simulink model "CF017A_GmVehPwrMod"  (R2013b)
settings: Solver=FixedStepDiscrete  SolverMode=SingleTasking  StartTime=0.0  StopTime=1  FixedStep=0.002  RelTol=1e-3
values from neighbouring files (symbols this model uses):
  ASSIKEEPMINIDX_CNT_U16 = DataDict.Constant    [CF017A_GmVehPwrMod_DataDict.m]
  BUSOFFHISPDIDX_CNT_U16 = DataDict.Constant    [CF017A_GmVehPwrMod_DataDict.m]
  CNTTOSEC_ULS_U32 = DataDict.Constant    [CF017A_GmVehPwrMod_DataDict.m]
  ENGRUNACTVIDX_CNT_U16 = DataDict.Constant    [CF017A_GmVehPwrMod_DataDict.m]
  GmVehPwrModHwTqMinKeepAssi = DataDict.Calibration    [CF017A_GmVehPwrMod_DataDict.m]
  GmVehPwrModHwTqMinKeepTmr = DataDict.Calibration    [CF017A_GmVehPwrMod_DataDict.m]
  GmVehPwrModOperRampRate = DataDict.Calibration    [CF017A_GmVehPwrMod_DataDict.m]
  GMVEHPWRMODSYSSTREQENA_CNT_LOGL = DataDict.Constant    [CF017A_GmVehPwrMod_DataDict.m]
  GMVEHPWRMODVAREFF_CNT_LOGL = DataDict.Constant    [CF017A_GmVehPwrMod_DataDict.m]
  GmVehPwrModVehSpdAssiOnMin = DataDict.Calibration    [CF017A_GmVehPwrMod_DataDict.m]
  GmVehPwrModVehSpdMinKeepAssi = DataDict.Calibration    [CF017A_GmVehPwrMod_DataDict.m]
  GPIOMCUENAIDX_CNT_U16 = DataDict.Constant    [CF017A_GmVehPwrMod_DataDict.m]
  KEEPASSIIDX_CNT_U16 = DataDict.Constant    [CF017A_GmVehPwrMod_DataDict.m]
  PRPNSYSACTVMSGINVLDIDX_CNT_U16 = DataDict.Constant    [CF017A_GmVehPwrMod_DataDict.m]
  SYSPWRMODMSGINVLDIDX_CNT_U16 = DataDict.Constant    [CF017A_GmVehPwrMod_DataDict.m]
  SYSPWRMODRUNIDX_CNT_U16 = DataDict.Constant    [CF017A_GmVehPwrMod_DataDict.m]
  VEHSPDSNSRVLDIDX_CNT_U16 = DataDict.Constant    [CF017A_GmVehPwrMod_DataDict.m]
libraries: simulink x2, NxtrLim x2, NxtrAbslt x1
(part 3 of 4)

== system CF017A_GmVehPwrMod/GmVehPwrMod/GmVehPwrModPer1/SysStReqEna_LookupTbl_KeepOn_OnToOff/EngRunActv_Bit6 ==
  In1 : Inport  RequirementInfo="{'linktype_rmi_doors' '0000c6e5 (/GM T1XX/SubSystem Specifications/Customer Functions/CF017A GM Vehicle Power Mode)' '#CF017A_114' 'true' 'REQ:  CF017A_114' '' } %GIDa_9dd018ca_3e31_4c4a_90e0_a6ac76f1343b"
  Bit6_0 : Subsystem  RequirementInfo="{'linktype_rmi_doors' '0000c6e5 (/GM T1XX/SubSystem Specifications/Customer Functions/CF017A GM Vehicle Power Mode)' '#CF017A_114' 'true' 'REQ:  CF017A_114' '' } %GIDa_625130ff_287d_43aa_9d60_330dce0521fa"  TreatAsAtomicUnit=on
  Bit6_64 : Subsystem  RequirementInfo="{'linktype_rmi_doors' '0000c6e5 (/GM T1XX/SubSystem Specifications/Customer Functions/CF017A GM Vehicle Power Mode)' '#CF017A_114' 'true' 'REQ:  CF017A_114' '' } %GIDa_af33270b_28d4_422a_b500_86faa96af759"  TreatAsAtomicUnit=on
  CopyRight2 : Subsystem  Description=|  mask(Copyright Information){none=on}
      | Copyright info block.                                               
      |                                                                     
      | Place copyright information at the top of every subsystem in design.
      mask prompts: none "No parameters"
      mask help: Place copyright information at the top of every subsystem in design.
      mask Display:
      | NxtrConf = 'Nexteer Confidential';
      | 
      | sys = bdroot; %handle for the current model ("system")
      | first = get_param(sys,'Created');
      | if(isempty(first))
      |     first = datestr(now,'yyyy');
      | else
      |     first = first(end-3:end);  %year is last four digits
      | end
      | 
      | last = get_param(sys,'LastModifiedDate');
      | if isempty(last)
      |     last = datestr(now,'yyyy');
      | else
      |     last = last(end-3:end);
      | end
      | 
      | if strcmp(first,last)
      |     fprintf('%s -- Copyright %s Nexteer',NxtrConf,first)
      | else
      |     fprintf('%s -- %s%s- %s Nexteer',NxtrConf,char(169),first,last)
      | end
  EngRunActv_IF : If  RequirementInfo="{'linktype_rmi_doors' '0000c6e5 (/GM T1XX/SubSystem Specifications/Customer Functions/CF017A GM Vehicle Power Mode)' '#CF017A_114' 'true' 'REQ:  CF017A_114' '' } %GIDa_4bc83484_183b_4007_801b_23b2c8241593"  IfExpression=u1
  Merge2 : Merge  RequirementInfo="{'linktype_rmi_doors' '0000c6e5 (/GM T1XX/SubSystem Specifications/Customer Functions/CF017A GM Vehicle Power Mode)' '#CF017A_114' 'true' 'REQ:  CF017A_114' '' } %GIDa_7048c8b7_9ac1_4109_96fa_021c302b5bde"
  Out1 : Outport  RequirementInfo="{'linktype_rmi_doors' '0000c6e5 (/GM T1XX/SubSystem Specifications/Customer Functions/CF017A GM Vehicle Power Mode)' '#CF017A_114' 'true' 'REQ:  CF017A_114' '' } %GIDa_5ffbc119_3c40_4564_a8d9_386f6fb67804"
  wires:
  In1/1 -> EngRunActv_IF/1
  EngRunActv_IF/1 -> Bit6_64/Action
  EngRunActv_IF/2 -> Bit6_0/Action
  Bit6_64/1(Bit6Sts) -> Merge2/1
  Bit6_0/1(Bit6Sts) -> Merge2/2
  Merge2/1 -> Out1/1

== system CF017A_GmVehPwrMod/GmVehPwrMod/GmVehPwrModPer1/SysStReqEna_LookupTbl_KeepOn_OnToOff/GpioMcuEna_Bit8 ==
  In : Inport  RequirementInfo="{'linktype_rmi_doors' '0000c6e5 (/GM T1XX/SubSystem Specifications/Customer Functions/CF017A GM Vehicle Power Mode)' '#CF017A_114' 'true' 'REQ:  CF017A_114' '' } %GIDa_b2d8aade_f5d0_444a_a063_7a0289bf908d"
  Bit8_0 : Subsystem  RequirementInfo="{'linktype_rmi_doors' '0000c6e5 (/GM T1XX/SubSystem Specifications/Customer Functions/CF017A GM Vehicle Power Mode)' '#CF017A_114' 'true' 'REQ:  CF017A_114' '' } %GIDa_98c494f0_6c2c_4ada_a798_589724dbf92f"  TreatAsAtomicUnit=on
  Bit8_256 : Subsystem  RequirementInfo="{'linktype_rmi_doors' '0000c6e5 (/GM T1XX/SubSystem Specifications/Customer Functions/CF017A GM Vehicle Power Mode)' '#CF017A_114' 'true' 'REQ:  CF017A_114' '' } %GIDa_a5e75daa_1c3b_4b0f_b862_b737ac528363"  TreatAsAtomicUnit=on
  CopyRight2 : Subsystem  Description=|  mask(Copyright Information){none=on}
      | Copyright info block.                                               
      |                                                                     
      | Place copyright information at the top of every subsystem in design.
      mask prompts: none "No parameters"
      mask help: Place copyright information at the top of every subsystem in design.
      mask Display:
      | NxtrConf = 'Nexteer Confidential';
      | 
      | sys = bdroot; %handle for the current model ("system")
      | first = get_param(sys,'Created');
      | if(isempty(first))
      |     first = datestr(now,'yyyy');
      | else
      |     first = first(end-3:end);  %year is last four digits
      | end
      | 
      | last = get_param(sys,'LastModifiedDate');
      | if isempty(last)
      |     last = datestr(now,'yyyy');
      | else
      |     last = last(end-3:end);
      | end
      | 
      | if strcmp(first,last)
      |     fprintf('%s -- Copyright %s Nexteer',NxtrConf,first)
      | else
      |     fprintf('%s -- %s%s- %s Nexteer',NxtrConf,char(169),first,last)
      | end
  GpioMcuEna_IF : If  RequirementInfo="{'linktype_rmi_doors' '0000c6e5 (/GM T1XX/SubSystem Specifications/Customer Functions/CF017A GM Vehicle Power Mode)' '#CF017A_114' 'true' 'REQ:  CF017A_114' '' } %GIDa_c15d6b31_07d4_4da5_92f4_eebbb80e631b"  IfExpression=u1
  Merge : Merge  RequirementInfo="{'linktype_rmi_doors' '0000c6e5 (/GM T1XX/SubSystem Specifications/Customer Functions/CF017A GM Vehicle Power Mode)' '#CF017A_114' 'true' 'REQ:  CF017A_114' '' } %GIDa_7ac9840a_6a47_4d26_9edd_f2dafb33ce57"
  Out : Outport  RequirementInfo="{'linktype_rmi_doors' '0000c6e5 (/GM T1XX/SubSystem Specifications/Customer Functions/CF017A GM Vehicle Power Mode)' '#CF017A_114' 'true' 'REQ:  CF017A_114' '' } %GIDa_ea86f811_2d4e_4aa3_b284_a4169a7d690f"
  wires:
  In/1 -> GpioMcuEna_IF/1
  GpioMcuEna_IF/1 -> Bit8_256/Action
  GpioMcuEna_IF/2 -> Bit8_0/Action
  Bit8_256/1(Bit8Sts) -> Merge/1
  Bit8_0/1(Bit8Sts) -> Merge/2
  Merge/1 -> Out/1

== system CF017A_GmVehPwrMod/GmVehPwrMod/GmVehPwrModPer1/SysStReqEna_LookupTbl_KeepOn_OnToOff/KeepAssi_Bit0 ==
  In1 : Inport  RequirementInfo="{'linktype_rmi_doors' '0000c6e5 (/GM T1XX/SubSystem Specifications/Customer Functions/CF017A GM Vehicle Power Mode)' '#CF017A_114' 'true' 'REQ:  CF017A_114' '' } %GIDa_256cbed8_1791_4f67_b60a_bd14ae39a67f"
  Bit0_0 : Subsystem  RequirementInfo="{'linktype_rmi_doors' '0000c6e5 (/GM T1XX/SubSystem Specifications/Customer Functions/CF017A GM Vehicle Power Mode)' '#CF017A_114' 'true' 'REQ:  CF017A_114' '' } %GIDa_151fd744_2109_4663_a40c_7bcc314cfd30"  TreatAsAtomicUnit=on
  Bit0_1 : Subsystem  RequirementInfo="{'linktype_rmi_doors' '0000c6e5 (/GM T1XX/SubSystem Specifications/Customer Functions/CF017A GM Vehicle Power Mode)' '#CF017A_114' 'true' 'REQ:  CF017A_114' '' } %GIDa_d6091671_229f_4d66_b3ca_8a783b9b5da7"  TreatAsAtomicUnit=on
  CopyRight2 : Subsystem  Description=|  mask(Copyright Information){none=on}
      | Copyright info block.                                               
      |                                                                     
      | Place copyright information at the top of every subsystem in design.
      mask prompts: none "No parameters"
      mask help: Place copyright information at the top of every subsystem in design.
      mask Display:
      | NxtrConf = 'Nexteer Confidential';
      | 
      | sys = bdroot; %handle for the current model ("system")
      | first = get_param(sys,'Created');
      | if(isempty(first))
      |     first = datestr(now,'yyyy');
      | else
      |     first = first(end-3:end);  %year is last four digits
      | end
      | 
      | last = get_param(sys,'LastModifiedDate');
      | if isempty(last)
      |     last = datestr(now,'yyyy');
      | else
      |     last = last(end-3:end);
      | end
      | 
      | if strcmp(first,last)
      |     fprintf('%s -- Copyright %s Nexteer',NxtrConf,first)
      | else
      |     fprintf('%s -- %s%s- %s Nexteer',NxtrConf,char(169),first,last)
      | end
  KeepAssi_IF : If  RequirementInfo="{'linktype_rmi_doors' '0000c6e5 (/GM T1XX/SubSystem Specifications/Customer Functions/CF017A GM Vehicle Power Mode)' '#CF017A_114' 'true' 'REQ:  CF017A_114' '' } %GIDa_0f92cfb0_47d9_40b4_bb82_e6a253e207e0"  IfExpression=u1
  Merge8 : Merge  RequirementInfo="{'linktype_rmi_doors' '0000c6e5 (/GM T1XX/SubSystem Specifications/Customer Functions/CF017A GM Vehicle Power Mode)' '#CF017A_114' 'true' 'REQ:  CF017A_114' '' } %GIDa_b6c3a93d_a990_4701_9ba0_c730f119e17e"
  Out1 : Outport  RequirementInfo="{'linktype_rmi_doors' '0000c6e5 (/GM T1XX/SubSystem Specifications/Customer Functions/CF017A GM Vehicle Power Mode)' '#CF017A_114' 'true' 'REQ:  CF017A_114' '' } %GIDa_34eb3cf8_5e70_447c_85ff_e4f5d4d1e942"
  wires:
  KeepAssi_IF/1 -> Bit0_1/Action
  KeepAssi_IF/2 -> Bit0_0/Action
  Bit0_1/1(Bit0Sts) -> Merge8/1
  Bit0_0/1(Bit0Sts) -> Merge8/2
  Merge8/1 -> Out1/1
  In1/1 -> KeepAssi_IF/1

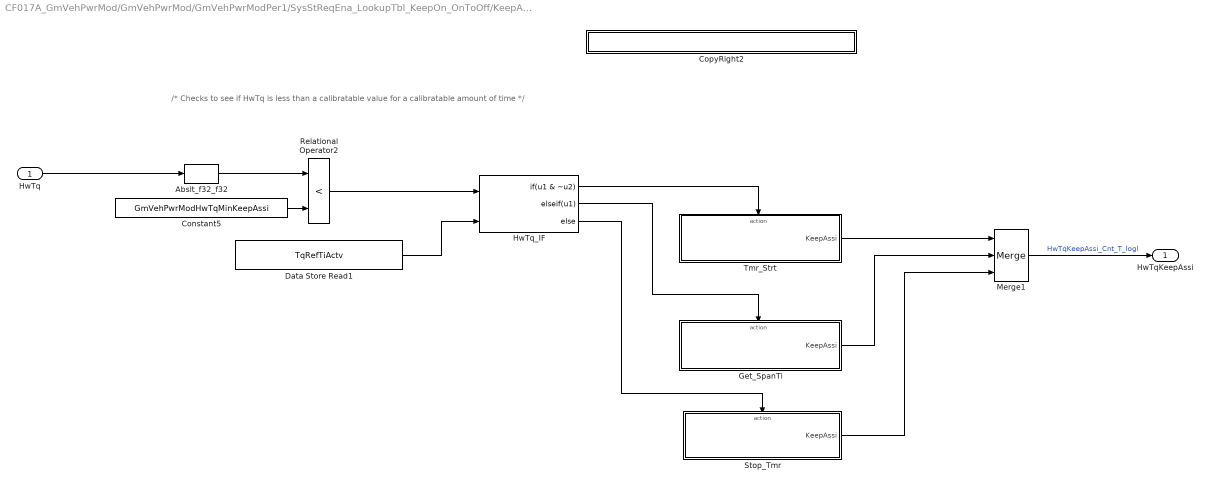
== system CF017A_GmVehPwrMod/GmVehPwrMod/GmVehPwrModPer1/SysStReqEna_LookupTbl_KeepOn_OnToOff/KeepAssi_HwTqTmr ==
  note: /* Checks to see if HwTq is less than a calibratable value for a calibratable amount of time */
  HwTq : Inport  RequirementInfo="{'linktype_rmi_doors' '0000c6e5 (/GM T1XX/SubSystem Specifications/Customer Functions/CF017A GM Vehicle Power Mode)' '#CF017A_114' 'true' 'REQ:  CF017A_114' '' } %GIDa_c3a6937b_df32_440c_ba95_13f74061466f"
  Abslt_f32_f32 : NxtrAbslt/Abslt_f32_f32  RequirementInfo="{'linktype_rmi_doors' '0000c6e5 (/GM T1XX/SubSystem Specifications/Customer Functions/CF017A GM Vehicle Power Mode)' '#CF017A_114' 'true' 'REQ:  CF017A_114' '' } %GIDa_3a5ba81e_d107_4fba_8a7b_6e86486cebbe"  SFunctionSpec=single y1 = Abslt_f32_f32(single u1)
      settings: AttributesFormatString=%<Name>
  Constant5 : Constant  RequirementInfo="{'linktype_rmi_doors' '0000c6e5 (/GM T1XX/SubSystem Specifications/Customer Functions/CF017A GM Vehicle Power Mode)' '#CF017A_114' 'true' 'REQ:  CF017A_114' '' } %GIDa_adffab70_fd73_4ddb_9985_73770c18bc3f"  Value=GmVehPwrModHwTqMinKeepAssi  OutDataTypeStr=single
      settings: AttributesFormatString=%<OutDataTypeStr>
  CopyRight2 : Subsystem  Description=|  mask(Copyright Information){none=on}
      | Copyright info block.                                               
      |                                                                     
      | Place copyright information at the top of every subsystem in design.
      mask prompts: none "No parameters"
      mask help: Place copyright information at the top of every subsystem in design.
      mask Display:
      | NxtrConf = 'Nexteer Confidential';
      | 
      | sys = bdroot; %handle for the current model ("system")
      | first = get_param(sys,'Created');
      | if(isempty(first))
      |     first = datestr(now,'yyyy');
      | else
      |     first = first(end-3:end);  %year is last four digits
      | end
      | 
      | last = get_param(sys,'LastModifiedDate');
      | if isempty(last)
      |     last = datestr(now,'yyyy');
      | else
      |     last = last(end-3:end);
      | end
      | 
      | if strcmp(first,last)
      |     fprintf('%s -- Copyright %s Nexteer',NxtrConf,first)
      | else
      |     fprintf('%s -- %s%s- %s Nexteer',NxtrConf,char(169),first,last)
      | end
  Data Store Read1 : DataStoreRead  RequirementInfo="{'linktype_rmi_doors' '0000c6e5 (/GM T1XX/SubSystem Specifications/Customer Functions/CF017A GM Vehicle Power Mode)' '#CF017A_114' 'true' 'REQ:  CF017A_114' '' } %GIDa_ae007e7c_6e91_4274_8f03_1bad8648c8eb"  DataStoreName=TqRefTiActv
  Get_SpanTi : Subsystem  RequirementInfo="{'linktype_rmi_doors' '0000c6e5 (/GM T1XX/SubSystem Specifications/Customer Functions/CF017A GM Vehicle Power Mode)' '#CF017A_114' 'true' 'REQ:  CF017A_114' '' } %GIDa_763799e1_0442_4180_996d_ddc443fffa17"  TreatAsAtomicUnit=on
  HwTq_IF : If  RequirementInfo="{'linktype_rmi_doors' '0000c6e5 (/GM T1XX/SubSystem Specifications/Customer Functions/CF017A GM Vehicle Power Mode)' '#CF017A_114' 'true' 'REQ:  CF017A_114' '' } %GIDa_62e46df0_927c_4046_91d3_c5bf11f90563"  NumInputs=2  IfExpression=u1 & ~u2  ElseIfExpressions=u1
      settings: AttributesFormatString=%<Priority>
  Merge1 : Merge  RequirementInfo="{'linktype_rmi_doors' '0000c6e5 (/GM T1XX/SubSystem Specifications/Customer Functions/CF017A GM Vehicle Power Mode)' '#CF017A_114' 'true' 'REQ:  CF017A_114' '' } %GIDa_e9a2ff01_7d75_46dd_8799_bdc1acdf7b88"  Inputs=3
  Relational Operator2 : RelationalOperator  RequirementInfo="{'linktype_rmi_doors' '0000c6e5 (/GM T1XX/SubSystem Specifications/Customer Functions/CF017A GM Vehicle Power Mode)' '#CF017A_114' 'true' 'REQ:  CF017A_114' '' } %GIDa_baf5e27b_ba36_44dd_ae20_e2eb1b2ebcf4"  Operator=<  OutDataTypeStr=boolean
  Stop_Tmr : Subsystem  RequirementInfo="{'linktype_rmi_doors' '0000c6e5 (/GM T1XX/SubSystem Specifications/Customer Functions/CF017A GM Vehicle Power Mode)' '#CF017A_114' 'true' 'REQ:  CF017A_114' '' } %GIDa_e3c3fd56_8c35_498f_9322_7430b0bab790"  TreatAsAtomicUnit=on
  Tmr_Strt : Subsystem  RequirementInfo="{'linktype_rmi_doors' '0000c6e5 (/GM T1XX/SubSystem Specifications/Customer Functions/CF017A GM Vehicle Power Mode)' '#CF017A_114' 'true' 'REQ:  CF017A_114' '' } %GIDa_1977e5b8_ee04_4209_b22f_32f27427e055"  TreatAsAtomicUnit=on
  HwTqKeepAssi : Outport  RequirementInfo="{'linktype_rmi_doors' '0000c6e5 (/GM T1XX/SubSystem Specifications/Customer Functions/CF017A GM Vehicle Power Mode)' '#CF017A_114' 'true' 'REQ:  CF017A_114' '' } %GIDa_e791da23_25c1_4c1a_9a17_68a71b1c395d"
  wires:
  Merge1/1 -> HwTqKeepAssi/1  "HwTqKeepAssi_Cnt_T_logl"
  HwTq/1 -> Abslt_f32_f32/1
  HwTq_IF/2 -> Get_SpanTi/Action
  Constant5/1 -> Relational Operator2/2
  Data Store Read1/1 -> HwTq_IF/2
  Abslt_f32_f32/1 -> Relational Operator2/1
  HwTq_IF/3 -> Stop_Tmr/Action
  Relational Operator2/1 -> HwTq_IF/1
  HwTq_IF/1 -> Tmr_Strt/Action
  Stop_Tmr/1("KeepAssi ") -> Merge1/3
  Tmr_Strt/1("KeepAssi ") -> Merge1/1
  Get_SpanTi/1("KeepAssi ") -> Merge1/2

== system CF017A_GmVehPwrMod/GmVehPwrMod/GmVehPwrModPer1/SysStReqEna_LookupTbl_KeepOn_OnToOff/PrpnSysActvMsgInvld_Bit4 ==
  In1 : Inport  RequirementInfo="{'linktype_rmi_doors' '0000c6e5 (/GM T1XX/SubSystem Specifications/Customer Functions/CF017A GM Vehicle Power Mode)' '#CF017A_114' 'true' 'REQ:  CF017A_114' '' } %GIDa_2c591430_5888_4c70_8e6c_3841059961a6"
  Bit4_0 : Subsystem  RequirementInfo="{'linktype_rmi_doors' '0000c6e5 (/GM T1XX/SubSystem Specifications/Customer Functions/CF017A GM Vehicle Power Mode)' '#CF017A_114' 'true' 'REQ:  CF017A_114' '' } %GIDa_0caf3abd_580a_4ffc_a4a2_093dd0efe2b5"  TreatAsAtomicUnit=on
  Bit4_16 : Subsystem  RequirementInfo="{'linktype_rmi_doors' '0000c6e5 (/GM T1XX/SubSystem Specifications/Customer Functions/CF017A GM Vehicle Power Mode)' '#CF017A_114' 'true' 'REQ:  CF017A_114' '' } %GIDa_14718cb4_63e4_496f_b47b_8227a685ab2f"  TreatAsAtomicUnit=on
  CopyRight2 : Subsystem  Description=|  mask(Copyright Information){none=on}
      | Copyright info block.                                               
      |                                                                     
      | Place copyright information at the top of every subsystem in design.
      mask prompts: none "No parameters"
      mask help: Place copyright information at the top of every subsystem in design.
      mask Display:
      | NxtrConf = 'Nexteer Confidential';
      | 
      | sys = bdroot; %handle for the current model ("system")
      | first = get_param(sys,'Created');
      | if(isempty(first))
      |     first = datestr(now,'yyyy');
      | else
      |     first = first(end-3:end);  %year is last four digits
      | end
      | 
      | last = get_param(sys,'LastModifiedDate');
      | if isempty(last)
      |     last = datestr(now,'yyyy');
      | else
      |     last = last(end-3:end);
      | end
      | 
      | if strcmp(first,last)
      |     fprintf('%s -- Copyright %s Nexteer',NxtrConf,first)
      | else
      |     fprintf('%s -- %s%s- %s Nexteer',NxtrConf,char(169),first,last)
      | end
  Merge4 : Merge  RequirementInfo="{'linktype_rmi_doors' '0000c6e5 (/GM T1XX/SubSystem Specifications/Customer Functions/CF017A GM Vehicle Power Mode)' '#CF017A_114' 'true' 'REQ:  CF017A_114' '' } %GIDa_4aefb7ab_6048_4fba_b30f_165c5c5a5fc7"
  Msg0C9Missa_IF : If  RequirementInfo="{'linktype_rmi_doors' '0000c6e5 (/GM T1XX/SubSystem Specifications/Customer Functions/CF017A GM Vehicle Power Mode)' '#CF017A_114' 'true' 'REQ:  CF017A_114' '' } %GIDa_4ef6b54c_1cdc_4af6_96da_f9013792689e"  IfExpression=u1
  Out1 : Outport  RequirementInfo="{'linktype_rmi_doors' '0000c6e5 (/GM T1XX/SubSystem Specifications/Customer Functions/CF017A GM Vehicle Power Mode)' '#CF017A_114' 'true' 'REQ:  CF017A_114' '' } %GIDa_0572da8d_4d01_4630_a2fe_8cdb88bfe4d3"
  wires:
  In1/1 -> Msg0C9Missa_IF/1
  Msg0C9Missa_IF/1 -> Bit4_16/Action
  Msg0C9Missa_IF/2 -> Bit4_0/Action
  Bit4_16/1(Bit4Sts) -> Merge4/1
  Bit4_0/1(Bit4Sts) -> Merge4/2
  Merge4/1 -> Out1/1

== system CF017A_GmVehPwrMod/GmVehPwrMod/GmVehPwrModPer1/SysStReqEna_LookupTbl_KeepOn_OnToOff/SysPwrModMsgInvld_Bit2 ==
  In1 : Inport  RequirementInfo="{'linktype_rmi_doors' '0000c6e5 (/GM T1XX/SubSystem Specifications/Customer Functions/CF017A GM Vehicle Power Mode)' '#CF017A_114' 'true' 'REQ:  CF017A_114' '' } %GIDa_b9b4edaa_6008_4e55_867c_388323464606"
  Bit2_0 : Subsystem  RequirementInfo="{'linktype_rmi_doors' '0000c6e5 (/GM T1XX/SubSystem Specifications/Customer Functions/CF017A GM Vehicle Power Mode)' '#CF017A_114' 'true' 'REQ:  CF017A_114' '' } %GIDa_b11557df_5945_49a6_a0af_1b2573475ba6"  TreatAsAtomicUnit=on
  Bit2_4 : Subsystem  RequirementInfo="{'linktype_rmi_doors' '0000c6e5 (/GM T1XX/SubSystem Specifications/Customer Functions/CF017A GM Vehicle Power Mode)' '#CF017A_114' 'true' 'REQ:  CF017A_114' '' } %GIDa_538bca24_1df9_41e8_ac8e_fc9e4c129984"  TreatAsAtomicUnit=on
  CopyRight2 : Subsystem  Description=|  mask(Copyright Information){none=on}
      | Copyright info block.                                               
      |                                                                     
      | Place copyright information at the top of every subsystem in design.
      mask prompts: none "No parameters"
      mask help: Place copyright information at the top of every subsystem in design.
      mask Display:
      | NxtrConf = 'Nexteer Confidential';
      | 
      | sys = bdroot; %handle for the current model ("system")
      | first = get_param(sys,'Created');
      | if(isempty(first))
      |     first = datestr(now,'yyyy');
      | else
      |     first = first(end-3:end);  %year is last four digits
      | end
      | 
      | last = get_param(sys,'LastModifiedDate');
      | if isempty(last)
      |     last = datestr(now,'yyyy');
      | else
      |     last = last(end-3:end);
      | end
      | 
      | if strcmp(first,last)
      |     fprintf('%s -- Copyright %s Nexteer',NxtrConf,first)
      | else
      |     fprintf('%s -- %s%s- %s Nexteer',NxtrConf,char(169),first,last)
      | end
  Merge6 : Merge  RequirementInfo="{'linktype_rmi_doors' '0000c6e5 (/GM T1XX/SubSystem Specifications/Customer Functions/CF017A GM Vehicle Power Mode)' '#CF017A_114' 'true' 'REQ:  CF017A_114' '' } %GIDa_c748d9e6_4e3c_4f18_8982_64515a3432db"
  Msg1F1Miss_IF : If  RequirementInfo="{'linktype_rmi_doors' '0000c6e5 (/GM T1XX/SubSystem Specifications/Customer Functions/CF017A GM Vehicle Power Mode)' '#CF017A_114' 'true' 'REQ:  CF017A_114' '' } %GIDa_7c507352_f8cc_4c21_a6de_4c1245659dbe"  IfExpression=u1
  Out1 : Outport  RequirementInfo="{'linktype_rmi_doors' '0000c6e5 (/GM T1XX/SubSystem Specifications/Customer Functions/CF017A GM Vehicle Power Mode)' '#CF017A_114' 'true' 'REQ:  CF017A_114' '' } %GIDa_11135a2a_4b33_4b18_b28c_32efa3fd628e"
  wires:
  In1/1 -> Msg1F1Miss_IF/1
  Msg1F1Miss_IF/1 -> Bit2_4/Action
  Msg1F1Miss_IF/2 -> Bit2_0/Action
  Bit2_4/1(Bit2Sts) -> Merge6/1
  Bit2_0/1(Bit2Sts) -> Merge6/2
  Merge6/1 -> Out1/1

== system CF017A_GmVehPwrMod/GmVehPwrMod/GmVehPwrModPer1/SysStReqEna_LookupTbl_KeepOn_OnToOff/SysPwrModRun_Bit7 ==
  In1 : Inport  RequirementInfo="{'linktype_rmi_doors' '0000c6e5 (/GM T1XX/SubSystem Specifications/Customer Functions/CF017A GM Vehicle Power Mode)' '#CF017A_114' 'true' 'REQ:  CF017A_114' '' } %GIDa_c1bc1cd8_ea72_4c59_9135_af5cdd5d310f"
  Bit7_0 : Subsystem  RequirementInfo="{'linktype_rmi_doors' '0000c6e5 (/GM T1XX/SubSystem Specifications/Customer Functions/CF017A GM Vehicle Power Mode)' '#CF017A_114' 'true' 'REQ:  CF017A_114' '' } %GIDa_c8c3ffe3_12b8_4e4f_8a91_02b5fec5e3dd"  TreatAsAtomicUnit=on
  Bit7_128 : Subsystem  RequirementInfo="{'linktype_rmi_doors' '0000c6e5 (/GM T1XX/SubSystem Specifications/Customer Functions/CF017A GM Vehicle Power Mode)' '#CF017A_114' 'true' 'REQ:  CF017A_114' '' } %GIDa_e75e24b2_0a88_446a_a5f8_10565f6eaf7b"  TreatAsAtomicUnit=on
  CopyRight2 : Subsystem  Description=|  mask(Copyright Information){none=on}
      | Copyright info block.                                               
      |                                                                     
      | Place copyright information at the top of every subsystem in design.
      mask prompts: none "No parameters"
      mask help: Place copyright information at the top of every subsystem in design.
      mask Display:
      | NxtrConf = 'Nexteer Confidential';
      | 
      | sys = bdroot; %handle for the current model ("system")
      | first = get_param(sys,'Created');
      | if(isempty(first))
      |     first = datestr(now,'yyyy');
      | else
      |     first = first(end-3:end);  %year is last four digits
      | end
      | 
      | last = get_param(sys,'LastModifiedDate');
      | if isempty(last)
      |     last = datestr(now,'yyyy');
      | else
      |     last = last(end-3:end);
      | end
      | 
      | if strcmp(first,last)
      |     fprintf('%s -- Copyright %s Nexteer',NxtrConf,first)
      | else
      |     fprintf('%s -- %s%s- %s Nexteer',NxtrConf,char(169),first,last)
      | end
  Merge1 : Merge  RequirementInfo="{'linktype_rmi_doors' '0000c6e5 (/GM T1XX/SubSystem Specifications/Customer Functions/CF017A GM Vehicle Power Mode)' '#CF017A_114' 'true' 'REQ:  CF017A_114' '' } %GIDa_47a35ad3_3413_4261_bf5c_ed15bdd468af"
  SysPwrModRun_IF : If  RequirementInfo="{'linktype_rmi_doors' '0000c6e5 (/GM T1XX/SubSystem Specifications/Customer Functions/CF017A GM Vehicle Power Mode)' '#CF017A_114' 'true' 'REQ:  CF017A_114' '' } %GIDa_3041b7fe_d5e9_45a7_907b_deaf3c12d1b7"  IfExpression=u1
  Out1 : Outport  RequirementInfo="{'linktype_rmi_doors' '0000c6e5 (/GM T1XX/SubSystem Specifications/Customer Functions/CF017A GM Vehicle Power Mode)' '#CF017A_114' 'true' 'REQ:  CF017A_114' '' } %GIDa_ea562539_c8ee_4d74_8941_942a4f0ad269"
  wires:
  In1/1 -> SysPwrModRun_IF/1
  SysPwrModRun_IF/1 -> Bit7_128/Action
  SysPwrModRun_IF/2 -> Bit7_0/Action
  Bit7_128/1(Bit7Sts) -> Merge1/1
  Bit7_0/1(Bit7Sts) -> Merge1/2
  Merge1/1 -> Out1/1

== system CF017A_GmVehPwrMod/GmVehPwrMod/GmVehPwrModPer1/SysStReqEna_LookupTbl_KeepOn_OnToOff/VehSpdSnsrVld_Bit3 ==
  In1 : Inport  RequirementInfo="{'linktype_rmi_doors' '0000c6e5 (/GM T1XX/SubSystem Specifications/Customer Functions/CF017A GM Vehicle Power Mode)' '#CF017A_114' 'true' 'REQ:  CF017A_114' '' } %GIDa_8aa9f388_a059_4463_8363_1874a8a11e12"
  Bit3_0 : Subsystem  RequirementInfo="{'linktype_rmi_doors' '0000c6e5 (/GM T1XX/SubSystem Specifications/Customer Functions/CF017A GM Vehicle Power Mode)' '#CF017A_114' 'true' 'REQ:  CF017A_114' '' } %GIDa_7ba2b7bb_b741_42b3_bd80_f659c1994e0e"  TreatAsAtomicUnit=on
  Bit3_8 : Subsystem  RequirementInfo="{'linktype_rmi_doors' '0000c6e5 (/GM T1XX/SubSystem Specifications/Customer Functions/CF017A GM Vehicle Power Mode)' '#CF017A_114' 'true' 'REQ:  CF017A_114' '' } %GIDa_fcf82675_d7c2_47d8_9612_37435f26f06f"  TreatAsAtomicUnit=on
  CopyRight2 : Subsystem  Description=|  mask(Copyright Information){none=on}
      | Copyright info block.                                               
      |                                                                     
      | Place copyright information at the top of every subsystem in design.
      mask prompts: none "No parameters"
      mask help: Place copyright information at the top of every subsystem in design.
      mask Display:
      | NxtrConf = 'Nexteer Confidential';
      | 
      | sys = bdroot; %handle for the current model ("system")
      | first = get_param(sys,'Created');
      | if(isempty(first))
      |     first = datestr(now,'yyyy');
      | else
      |     first = first(end-3:end);  %year is last four digits
      | end
      | 
      | last = get_param(sys,'LastModifiedDate');
      | if isempty(last)
      |     last = datestr(now,'yyyy');
      | else
      |     last = last(end-3:end);
      | end
      | 
      | if strcmp(first,last)
      |     fprintf('%s -- Copyright %s Nexteer',NxtrConf,first)
      | else
      |     fprintf('%s -- %s%s- %s Nexteer',NxtrConf,char(169),first,last)
      | end
  Merge5 : Merge  RequirementInfo="{'linktype_rmi_doors' '0000c6e5 (/GM T1XX/SubSystem Specifications/Customer Functions/CF017A GM Vehicle Power Mode)' '#CF017A_114' 'true' 'REQ:  CF017A_114' '' } %GIDa_5fe1fb49_98f0_4faf_b2eb_ad195c38c3fa"
  VehSpdSnsrVld_IF : If  RequirementInfo="{'linktype_rmi_doors' '0000c6e5 (/GM T1XX/SubSystem Specifications/Customer Functions/CF017A GM Vehicle Power Mode)' '#CF017A_114' 'true' 'REQ:  CF017A_114' '' } %GIDa_38f90319_4c08_4272_be31_7c36c1ecbd1c"  IfExpression=u1
  Out1 : Outport  RequirementInfo="{'linktype_rmi_doors' '0000c6e5 (/GM T1XX/SubSystem Specifications/Customer Functions/CF017A GM Vehicle Power Mode)' '#CF017A_114' 'true' 'REQ:  CF017A_114' '' } %GIDa_4d69da4a_8e85_4df4_ba86_5b3d7666622a"
  wires:
  In1/1 -> VehSpdSnsrVld_IF/1
  VehSpdSnsrVld_IF/1 -> Bit3_8/Action
  VehSpdSnsrVld_IF/2 -> Bit3_0/Action
  Bit3_8/1(Bit3Sts) -> Merge5/1
  Bit3_0/1(Bit3Sts) -> Merge5/2
  Merge5/1 -> Out1/1

== system CF017A_GmVehPwrMod/GmVehPwrMod/GmVehPwrModPer1/SysStReqEna_Ovrd/CopyRight2 ==

== system CF017A_GmVehPwrMod/GmVehPwrMod/GmVehPwrModPer1/TqCmdSca_VehSpdEna_Sub/CopyRight2 ==

== system CF017A_GmVehPwrMod/GmVehPwrMod/GmVehPwrModPer1/TqCmdSca_VehSpdEna_Sub/Set_SpdEna_False ==
  Action Port : ActionPort  ActionType=else
  Constant4 : Constant  RequirementInfo={} %GIDa_c969a244_c718_4e47_8c5d_d3e9949f60e3  Value=false  OutDataTypeStr=boolean
      settings: AttributesFormatString=%<OutDataTypeStr>
  CopyRight2 : Subsystem  Description=|  mask(Copyright Information){none=on}
      | Copyright info block.                                               
      |                                                                     
      | Place copyright information at the top of every subsystem in design.
      mask prompts: none "No parameters"
      mask help: Place copyright information at the top of every subsystem in design.
      mask Display:
      | NxtrConf = 'Nexteer Confidential';
      | 
      | sys = bdroot; %handle for the current model ("system")
      | first = get_param(sys,'Created');
      | if(isempty(first))
      |     first = datestr(now,'yyyy');
      | else
      |     first = first(end-3:end);  %year is last four digits
      | end
      | 
      | last = get_param(sys,'LastModifiedDate');
      | if isempty(last)
      |     last = datestr(now,'yyyy');
      | else
      |     last = last(end-3:end);
      | end
      | 
      | if strcmp(first,last)
      |     fprintf('%s -- Copyright %s Nexteer',NxtrConf,first)
      | else
      |     fprintf('%s -- %s%s- %s Nexteer',NxtrConf,char(169),first,last)
      | end
  "VehPwrModDftVehSpdEna " : Outport  RequirementInfo={} %GIDa_8e8bb61c_0665_4633_a294_c6f31ae58305
  wires:
  Constant4/1 -> "VehPwrModDftVehSpdEna "/1

== system CF017A_GmVehPwrMod/GmVehPwrMod/GmVehPwrModPer1/TqCmdSca_VehSpdEna_Sub/Set_SpdEna_True ==
  Action Port : ActionPort  ActionType=then
  Constant4 : Constant  RequirementInfo={} %GIDa_68d2d2ab_9cf3_4882_b287_021cb7e5d3a2  Value=true  OutDataTypeStr=boolean
      settings: AttributesFormatString=%<OutDataTypeStr>
  CopyRight2 : Subsystem  Description=|  mask(Copyright Information){none=on}
      | Copyright info block.                                               
      |                                                                     
      | Place copyright information at the top of every subsystem in design.
      mask prompts: none "No parameters"
      mask help: Place copyright information at the top of every subsystem in design.
      mask Display:
      | NxtrConf = 'Nexteer Confidential';
      | 
      | sys = bdroot; %handle for the current model ("system")
      | first = get_param(sys,'Created');
      | if(isempty(first))
      |     first = datestr(now,'yyyy');
      | else
      |     first = first(end-3:end);  %year is last four digits
      | end
      | 
      | last = get_param(sys,'LastModifiedDate');
      | if isempty(last)
      |     last = datestr(now,'yyyy');
      | else
      |     last = last(end-3:end);
      | end
      | 
      | if strcmp(first,last)
      |     fprintf('%s -- Copyright %s Nexteer',NxtrConf,first)
      | else
      |     fprintf('%s -- %s%s- %s Nexteer',NxtrConf,char(169),first,last)
      | end
  "VehPwrModDftVehSpdEna " : Outport  RequirementInfo={} %GIDa_cf3d7fa0_713b_4590_9a5a_32eeb1bd4bc9
  wires:
  Constant4/1 -> "VehPwrModDftVehSpdEna "/1

== system CF017A_GmVehPwrMod/GmVehPwrMod/GmVehPwrModPer1/TqCmdSca_VehSpdEna_Sub/TqCmdSca_0 ==
  Action Port : ActionPort  ActionType=else
  Constant3 : Constant  RequirementInfo="{'linktype_rmi_doors' '0000c6e5 (/GM T1XX/SubSystem Specifications/Customer Functions/CF017A GM Vehicle Power Mode)' '#CF017A_141' 'true' 'REQ:  CF017A_141' '' } %GIDa_6728cc2d_06c9_4a30_b7ce_581745178746"  Value=0  OutDataTypeStr=single
      settings: AttributesFormatString=%<OutDataTypeStr>
  CopyRight2 : Subsystem  Description=|  mask(Copyright Information){none=on}
      | Copyright info block.                                               
      |                                                                     
      | Place copyright information at the top of every subsystem in design.
      mask prompts: none "No parameters"
      mask help: Place copyright information at the top of every subsystem in design.
      mask Display:
      | NxtrConf = 'Nexteer Confidential';
      | 
      | sys = bdroot; %handle for the current model ("system")
      | first = get_param(sys,'Created');
      | if(isempty(first))
      |     first = datestr(now,'yyyy');
      | else
      |     first = first(end-3:end);  %year is last four digits
      | end
      | 
      | last = get_param(sys,'LastModifiedDate');
      | if isempty(last)
      |     last = datestr(now,'yyyy');
      | else
      |     last = last(end-3:end);
      | end
      | 
      | if strcmp(first,last)
      |     fprintf('%s -- Copyright %s Nexteer',NxtrConf,first)
      | else
      |     fprintf('%s -- %s%s- %s Nexteer',NxtrConf,char(169),first,last)
      | end
  SysOperMotTqCmdSca : Outport  RequirementInfo="{'linktype_rmi_doors' '0000c6e5 (/GM T1XX/SubSystem Specifications/Customer Functions/CF017A GM Vehicle Power Mode)' '#CF017A_141' 'true' 'REQ:  CF017A_141' '' } %GIDa_45580eef_5c3d_47bb_8207_d1896df57891"
  wires:
  Constant3/1 -> SysOperMotTqCmdSca/1

== system CF017A_GmVehPwrMod/GmVehPwrMod/GmVehPwrModPer1/TqCmdSca_VehSpdEna_Sub/TqCmdSca_1 ==
  Action Port : ActionPort  ActionType=then
  Constant3 : Constant  RequirementInfo="{'linktype_rmi_doors' '0000c6e5 (/GM T1XX/SubSystem Specifications/Customer Functions/CF017A GM Vehicle Power Mode)' '#CF017A_140' 'true' 'REQ:  CF017A_140' '' } %GIDa_de4d9e3c_2f27_4979_bc11_a6c27cecaf0c"  OutDataTypeStr=single
      settings: AttributesFormatString=%<OutDataTypeStr>
  CopyRight2 : Subsystem  Description=|  mask(Copyright Information){none=on}
      | Copyright info block.                                               
      |                                                                     
      | Place copyright information at the top of every subsystem in design.
      mask prompts: none "No parameters"
      mask help: Place copyright information at the top of every subsystem in design.
      mask Display:
      | NxtrConf = 'Nexteer Confidential';
      | 
      | sys = bdroot; %handle for the current model ("system")
      | first = get_param(sys,'Created');
      | if(isempty(first))
      |     first = datestr(now,'yyyy');
      | else
      |     first = first(end-3:end);  %year is last four digits
      | end
      | 
      | last = get_param(sys,'LastModifiedDate');
      | if isempty(last)
      |     last = datestr(now,'yyyy');
      | else
      |     last = last(end-3:end);
      | end
      | 
      | if strcmp(first,last)
      |     fprintf('%s -- Copyright %s Nexteer',NxtrConf,first)
      | else
      |     fprintf('%s -- %s%s- %s Nexteer',NxtrConf,char(169),first,last)
      | end
  SysOperMotTqCmdSca : Outport  RequirementInfo="{'linktype_rmi_doors' '0000c6e5 (/GM T1XX/SubSystem Specifications/Customer Functions/CF017A GM Vehicle Power Mode)' '#CF017A_140' 'true' 'REQ:  CF017A_140' '' } %GIDa_a7bc3936_d85d_4417_8c6d_43324766451b"
  wires:
  Constant3/1 -> SysOperMotTqCmdSca/1

== system CF017A_GmVehPwrMod/GmVehPwrMod/GmVehPwrModPer1/AssiOnMin_AssiKeepMin/AssiKeepMin_False/CopyRight2 ==

== system CF017A_GmVehPwrMod/GmVehPwrMod/GmVehPwrModPer1/AssiOnMin_AssiKeepMin/AssiKeepMin_True/CopyRight2 ==

== system CF017A_GmVehPwrMod/GmVehPwrMod/GmVehPwrModPer1/AssiOnMin_AssiKeepMin/AssiOnMin_False/CopyRight2 ==

== system CF017A_GmVehPwrMod/GmVehPwrMod/GmVehPwrModPer1/AssiOnMin_AssiKeepMin/AssiOnMin_True/CopyRight2 ==

== system CF017A_GmVehPwrMod/GmVehPwrMod/GmVehPwrModPer1/PwrSplyEnaReq_Sub/PwrSplyEnReq_False/CopyRight2 ==

== system CF017A_GmVehPwrMod/GmVehPwrMod/GmVehPwrModPer1/PwrSplyEnaReq_Sub/PwrSplyEnReq_True/CopyRight2 ==

== system CF017A_GmVehPwrMod/GmVehPwrMod/GmVehPwrModPer1/SysStReqEna_AssiOffToOn/Set_SysStReqEna_False/CopyRight2 ==

== system CF017A_GmVehPwrMod/GmVehPwrMod/GmVehPwrModPer1/SysStReqEna_AssiOffToOn/Set_SysStReqEna_True_Con1/CopyRight2 ==

== system CF017A_GmVehPwrMod/GmVehPwrMod/GmVehPwrModPer1/SysStReqEna_AssiOffToOn/Set_SysStReqEna_True_Con2/CopyRight2 ==

== system CF017A_GmVehPwrMod/GmVehPwrMod/GmVehPwrModPer1/SysStReqEna_LookupTbl_KeepOn_OnToOff/AssiKeepMin_Bit5/Bit5_0 ==
  Action Port : ActionPort  ActionType=else
  Constant2 : Constant  Value=0  OutDataTypeStr=uint16
      settings: AttributesFormatString=%<OutDataTypeStr>
  CopyRight2 : Subsystem  Description=|  mask(Copyright Information){none=on}
      | Copyright info block.                                               
      |                                                                     
      | Place copyright information at the top of every subsystem in design.
      mask prompts: none "No parameters"
      mask help: Place copyright information at the top of every subsystem in design.
      mask Display:
      | NxtrConf = 'Nexteer Confidential';
      | 
      | sys = bdroot; %handle for the current model ("system")
      | first = get_param(sys,'Created');
      | if(isempty(first))
      |     first = datestr(now,'yyyy');
      | else
      |     first = first(end-3:end);  %year is last four digits
      | end
      | 
      | last = get_param(sys,'LastModifiedDate');
      | if isempty(last)
      |     last = datestr(now,'yyyy');
      | else
      |     last = last(end-3:end);
      | end
      | 
      | if strcmp(first,last)
      |     fprintf('%s -- Copyright %s Nexteer',NxtrConf,first)
      | else
      |     fprintf('%s -- %s%s- %s Nexteer',NxtrConf,char(169),first,last)
      | end
  Bit5Sts : Outport
  wires:
  Constant2/1 -> Bit5Sts/1

== system CF017A_GmVehPwrMod/GmVehPwrMod/GmVehPwrModPer1/SysStReqEna_LookupTbl_KeepOn_OnToOff/AssiKeepMin_Bit5/Bit5_32 ==
  Action Port : ActionPort  ActionType=then
  Constant : Constant  Value=ASSIKEEPMINIDX_CNT_U16  OutDataTypeStr=uint16
  CopyRight2 : Subsystem  Description=|  mask(Copyright Information){none=on}
      | Copyright info block.                                               
      |                                                                     
      | Place copyright information at the top of every subsystem in design.
      mask prompts: none "No parameters"
      mask help: Place copyright information at the top of every subsystem in design.
      mask Display:
      | NxtrConf = 'Nexteer Confidential';
      | 
      | sys = bdroot; %handle for the current model ("system")
      | first = get_param(sys,'Created');
      | if(isempty(first))
      |     first = datestr(now,'yyyy');
      | else
      |     first = first(end-3:end);  %year is last four digits
      | end
      | 
      | last = get_param(sys,'LastModifiedDate');
      | if isempty(last)
      |     last = datestr(now,'yyyy');
      | else
      |     last = last(end-3:end);
      | end
      | 
      | if strcmp(first,last)
      |     fprintf('%s -- Copyright %s Nexteer',NxtrConf,first)
      | else
      |     fprintf('%s -- %s%s- %s Nexteer',NxtrConf,char(169),first,last)
      | end
  Bit5Sts : Outport
  wires:
  Constant/1 -> Bit5Sts/1

== system CF017A_GmVehPwrMod/GmVehPwrMod/GmVehPwrModPer1/SysStReqEna_LookupTbl_KeepOn_OnToOff/AssiKeepMin_Bit5/CopyRight2 ==

== system CF017A_GmVehPwrMod/GmVehPwrMod/GmVehPwrModPer1/SysStReqEna_LookupTbl_KeepOn_OnToOff/BusOffHiSpd_Bit1/Bit1_0 ==
  Action Port : ActionPort  ActionType=else
  Constant1 : Constant  Value=0  OutDataTypeStr=uint16
      settings: AttributesFormatString=%<OutDataTypeStr>
  CopyRight2 : Subsystem  Description=|  mask(Copyright Information){none=on}
      | Copyright info block.                                               
      |                                                                     
      | Place copyright information at the top of every subsystem in design.
      mask prompts: none "No parameters"
      mask help: Place copyright information at the top of every subsystem in design.
      mask Display:
      | NxtrConf = 'Nexteer Confidential';
      | 
      | sys = bdroot; %handle for the current model ("system")
      | first = get_param(sys,'Created');
      | if(isempty(first))
      |     first = datestr(now,'yyyy');
      | else
      |     first = first(end-3:end);  %year is last four digits
      | end
      | 
      | last = get_param(sys,'LastModifiedDate');
      | if isempty(last)
      |     last = datestr(now,'yyyy');
      | else
      |     last = last(end-3:end);
      | end
      | 
      | if strcmp(first,last)
      |     fprintf('%s -- Copyright %s Nexteer',NxtrConf,first)
      | else
      |     fprintf('%s -- %s%s- %s Nexteer',NxtrConf,char(169),first,last)
      | end
  Bit1Sts : Outport
  wires:
  Constant1/1 -> Bit1Sts/1

== system CF017A_GmVehPwrMod/GmVehPwrMod/GmVehPwrModPer1/SysStReqEna_LookupTbl_KeepOn_OnToOff/BusOffHiSpd_Bit1/Bit1_2 ==
  Action Port : ActionPort  ActionType=then
  Constant : Constant  Value=BUSOFFHISPDIDX_CNT_U16  OutDataTypeStr=uint16
  CopyRight2 : Subsystem  Description=|  mask(Copyright Information){none=on}
      | Copyright info block.                                               
      |                                                                     
      | Place copyright information at the top of every subsystem in design.
      mask prompts: none "No parameters"
      mask help: Place copyright information at the top of every subsystem in design.
      mask Display:
      | NxtrConf = 'Nexteer Confidential';
      | 
      | sys = bdroot; %handle for the current model ("system")
      | first = get_param(sys,'Created');
      | if(isempty(first))
      |     first = datestr(now,'yyyy');
      | else
      |     first = first(end-3:end);  %year is last four digits
      | end
      | 
      | last = get_param(sys,'LastModifiedDate');
      | if isempty(last)
      |     last = datestr(now,'yyyy');
      | else
      |     last = last(end-3:end);
      | end
      | 
      | if strcmp(first,last)
      |     fprintf('%s -- Copyright %s Nexteer',NxtrConf,first)
      | else
      |     fprintf('%s -- %s%s- %s Nexteer',NxtrConf,char(169),first,last)
      | end
  Bit1Sts : Outport
  wires:
  Constant/1 -> Bit1Sts/1

== system CF017A_GmVehPwrMod/GmVehPwrMod/GmVehPwrModPer1/SysStReqEna_LookupTbl_KeepOn_OnToOff/BusOffHiSpd_Bit1/CopyRight2 ==

== system CF017A_GmVehPwrMod/GmVehPwrMod/GmVehPwrModPer1/SysStReqEna_LookupTbl_KeepOn_OnToOff/EngRunActv_Bit6/Bit6_0 ==
  Action Port : ActionPort  ActionType=else
  Constant1 : Constant  Value=0  OutDataTypeStr=uint16
      settings: AttributesFormatString=%<OutDataTypeStr>
  CopyRight2 : Subsystem  Description=|  mask(Copyright Information){none=on}
      | Copyright info block.                                               
      |                                                                     
      | Place copyright information at the top of every subsystem in design.
      mask prompts: none "No parameters"
      mask help: Place copyright information at the top of every subsystem in design.
      mask Display:
      | NxtrConf = 'Nexteer Confidential';
      | 
      | sys = bdroot; %handle for the current model ("system")
      | first = get_param(sys,'Created');
      | if(isempty(first))
      |     first = datestr(now,'yyyy');
      | else
      |     first = first(end-3:end);  %year is last four digits
      | end
      | 
      | last = get_param(sys,'LastModifiedDate');
      | if isempty(last)
      |     last = datestr(now,'yyyy');
      | else
      |     last = last(end-3:end);
      | end
      | 
      | if strcmp(first,last)
      |     fprintf('%s -- Copyright %s Nexteer',NxtrConf,first)
      | else
      |     fprintf('%s -- %s%s- %s Nexteer',NxtrConf,char(169),first,last)
      | end
  Bit6Sts : Outport
  wires:
  Constant1/1 -> Bit6Sts/1

== system CF017A_GmVehPwrMod/GmVehPwrMod/GmVehPwrModPer1/SysStReqEna_LookupTbl_KeepOn_OnToOff/EngRunActv_Bit6/Bit6_64 ==
  Action Port : ActionPort  ActionType=then
  Constant : Constant  Value=ENGRUNACTVIDX_CNT_U16  OutDataTypeStr=uint16
  CopyRight2 : Subsystem  Description=|  mask(Copyright Information){none=on}
      | Copyright info block.                                               
      |                                                                     
      | Place copyright information at the top of every subsystem in design.
      mask prompts: none "No parameters"
      mask help: Place copyright information at the top of every subsystem in design.
      mask Display:
      | NxtrConf = 'Nexteer Confidential';
      | 
      | sys = bdroot; %handle for the current model ("system")
      | first = get_param(sys,'Created');
      | if(isempty(first))
      |     first = datestr(now,'yyyy');
      | else
      |     first = first(end-3:end);  %year is last four digits
      | end
      | 
      | last = get_param(sys,'LastModifiedDate');
      | if isempty(last)
      |     last = datestr(now,'yyyy');
      | else
      |     last = last(end-3:end);
      | end
      | 
      | if strcmp(first,last)
      |     fprintf('%s -- Copyright %s Nexteer',NxtrConf,first)
      | else
      |     fprintf('%s -- %s%s- %s Nexteer',NxtrConf,char(169),first,last)
      | end
  Bit6Sts : Outport
  wires:
  Constant/1 -> Bit6Sts/1

== system CF017A_GmVehPwrMod/GmVehPwrMod/GmVehPwrModPer1/SysStReqEna_LookupTbl_KeepOn_OnToOff/EngRunActv_Bit6/CopyRight2 ==

== system CF017A_GmVehPwrMod/GmVehPwrMod/GmVehPwrModPer1/SysStReqEna_LookupTbl_KeepOn_OnToOff/GpioMcuEna_Bit8/Bit8_0 ==
  Action Port : ActionPort  ActionType=else
  Constant1 : Constant  Value=0  OutDataTypeStr=uint16
      settings: AttributesFormatString=%<OutDataTypeStr>
  CopyRight2 : Subsystem  Description=|  mask(Copyright Information){none=on}
      | Copyright info block.                                               
      |                                                                     
      | Place copyright information at the top of every subsystem in design.
      mask prompts: none "No parameters"
      mask help: Place copyright information at the top of every subsystem in design.
      mask Display:
      | NxtrConf = 'Nexteer Confidential';
      | 
      | sys = bdroot; %handle for the current model ("system")
      | first = get_param(sys,'Created');
      | if(isempty(first))
      |     first = datestr(now,'yyyy');
      | else
      |     first = first(end-3:end);  %year is last four digits
      | end
      | 
      | last = get_param(sys,'LastModifiedDate');
      | if isempty(last)
      |     last = datestr(now,'yyyy');
      | else
      |     last = last(end-3:end);
      | end
      | 
      | if strcmp(first,last)
      |     fprintf('%s -- Copyright %s Nexteer',NxtrConf,first)
      | else
      |     fprintf('%s -- %s%s- %s Nexteer',NxtrConf,char(169),first,last)
      | end
  Bit8Sts : Outport
  wires:
  Constant1/1 -> Bit8Sts/1

== system CF017A_GmVehPwrMod/GmVehPwrMod/GmVehPwrModPer1/SysStReqEna_LookupTbl_KeepOn_OnToOff/GpioMcuEna_Bit8/Bit8_256 ==
  Action Port : ActionPort  ActionType=then
  Constant : Constant  Value=GPIOMCUENAIDX_CNT_U16  OutDataTypeStr=uint16
  CopyRight2 : Subsystem  Description=|  mask(Copyright Information){none=on}
      | Copyright info block.                                               
      |                                                                     
      | Place copyright information at the top of every subsystem in design.
      mask prompts: none "No parameters"
      mask help: Place copyright information at the top of every subsystem in design.
      mask Display:
      | NxtrConf = 'Nexteer Confidential';
      | 
      | sys = bdroot; %handle for the current model ("system")
      | first = get_param(sys,'Created');
      | if(isempty(first))
      |     first = datestr(now,'yyyy');
      | else
      |     first = first(end-3:end);  %year is last four digits
      | end
      | 
      | last = get_param(sys,'LastModifiedDate');
      | if isempty(last)
      |     last = datestr(now,'yyyy');
      | else
      |     last = last(end-3:end);
      | end
      | 
      | if strcmp(first,last)
      |     fprintf('%s -- Copyright %s Nexteer',NxtrConf,first)
      | else
      |     fprintf('%s -- %s%s- %s Nexteer',NxtrConf,char(169),first,last)
      | end
  Bit8Sts : Outport
  wires:
  Constant/1 -> Bit8Sts/1

== system CF017A_GmVehPwrMod/GmVehPwrMod/GmVehPwrModPer1/SysStReqEna_LookupTbl_KeepOn_OnToOff/GpioMcuEna_Bit8/CopyRight2 ==

== system CF017A_GmVehPwrMod/GmVehPwrMod/GmVehPwrModPer1/SysStReqEna_LookupTbl_KeepOn_OnToOff/KeepAssi_Bit0/Bit0_0 ==
  Action Port : ActionPort  ActionType=else
  Constant1 : Constant  Value=0  OutDataTypeStr=uint16
      settings: AttributesFormatString=%<OutDataTypeStr>
  CopyRight2 : Subsystem  Description=|  mask(Copyright Information){none=on}
      | Copyright info block.                                               
      |                                                                     
      | Place copyright information at the top of every subsystem in design.
      mask prompts: none "No parameters"
      mask help: Place copyright information at the top of every subsystem in design.
      mask Display:
      | NxtrConf = 'Nexteer Confidential';
      | 
      | sys = bdroot; %handle for the current model ("system")
      | first = get_param(sys,'Created');
      | if(isempty(first))
      |     first = datestr(now,'yyyy');
      | else
      |     first = first(end-3:end);  %year is last four digits
      | end
      | 
      | last = get_param(sys,'LastModifiedDate');
      | if isempty(last)
      |     last = datestr(now,'yyyy');
      | else
      |     last = last(end-3:end);
      | end
      | 
      | if strcmp(first,last)
      |     fprintf('%s -- Copyright %s Nexteer',NxtrConf,first)
      | else
      |     fprintf('%s -- %s%s- %s Nexteer',NxtrConf,char(169),first,last)
      | end
  Bit0Sts : Outport
  wires:
  Constant1/1 -> Bit0Sts/1
